simulink model "Simulation_3DOF"  (R2024a)
settings: Solver=ode4  StartTime=initial_time  StopTime=final_time  FixedStep=timestep  RelTol=1e-3
values from neighbouring files (symbols this model uses):
  gamma = 1.4    [Constants_3DOF.m]
  mass = 161.5    [Constants_3DOF.m]
  mu_earth = 3.986004418 * 10^14    (= 398600441800000)    [Constants_3DOF.m]
  r_earth = 6371.0088 * 10^3    (= 6371008.8)    [Constants_3DOF.m]
  wing_area = 0.079813    [Constants_3DOF.m]
undefined symbols (not defined in the file or in its folder): alpha, beta, c_d, c_l, rho, thrust, velocity, x, y, z
settings Model: Creator=641893  LastModifiedBy=641893

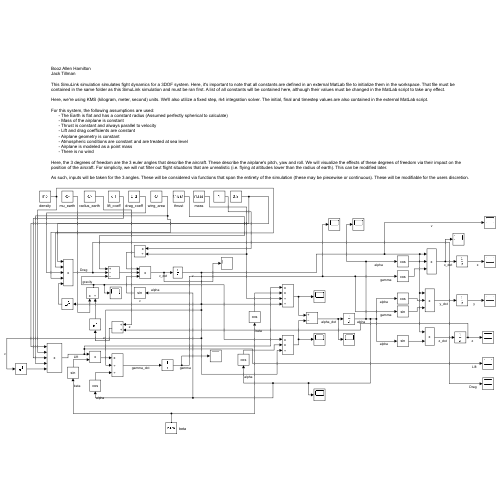
[thumbnail: Simulink's stored preview of the top-level diagram]
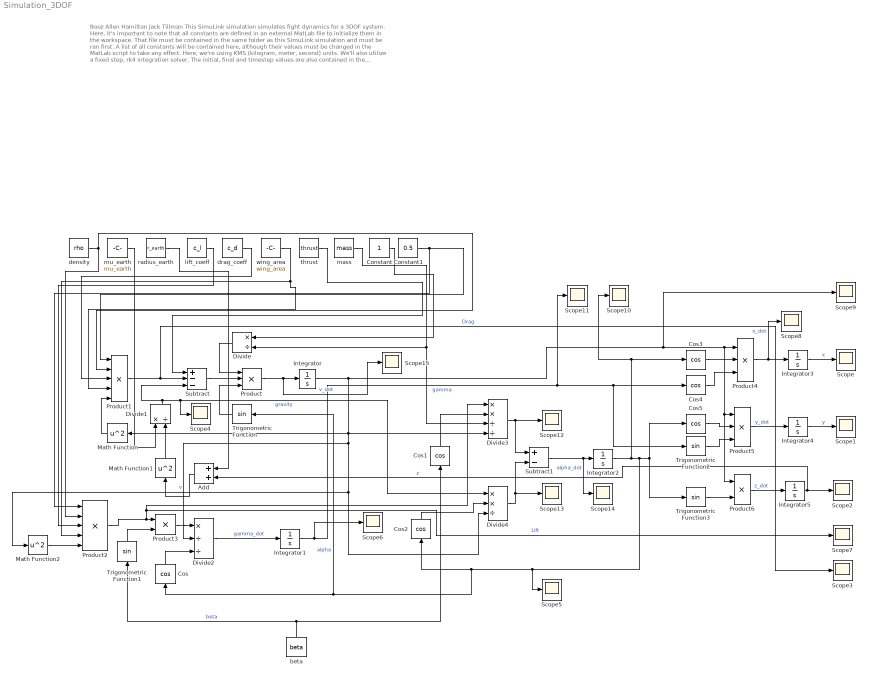
== system Simulation_3DOF ==
  note: Booz Allen Hamilton
      | Jack Tillman
      |
      | This SimuLink simulation simulates fight dynamics for a 3DOF system. Here, it's important to note that all constants are defined in an external MatLab file to initialize them in the workspace. That file must be contained in the same folder as this SimuLink simulation and must be ran first. A list of all constants will be contained here, although their values must be changed in the MatLab script to take any effect.
      |
      | Here, we're using KMS (kilogram, meter, second) units. We'll also utilize a fixed step, rk4 integration solver. The initial, final and timestep values are also contained in the external MatLab script.
      |
      | For this system, the following assumptions are used:
      | - The Earth is flat and has a constant radius (Assumed perfectly spherical to calculate)
      | - Mass of the airplane is constant
      | - Thrust is constant and always parallel to velocity
      | - Lift and drag coefficients are constant
      | - Airplane geometry is constant
      | - Atmospheric conditions are constant and are treated at sea level
      | - Airplane is modeled as a point mass
      | - There is no wind
      |
      | Here, the 3 degrees of freedom are the 3 euler angles that describe the aircraft. These describe the airplane's pitch, yaw and roll. We will visualize the effects of these degrees of freedom via their impact on the position of the aircraft. For simplicity, we will not filter out flight situations that are unrealistic (i.e. flying at altitudes lower than the radius of earth). This can be modified later.
      |
      | As such, inputs will be taken for the 3 angles. These will be considered via functions that span the entirety of the simulation (these may be piecewise or continuous). These will be modifiable for the users discretion.
  Add : Sum
  Constant : Constant
  Constant1 : Constant  Value=0.5
  Cos{,1..5} (6 alike) : Trigonometry  Operator=cos
  Divide : Product  Inputs=*/
  Divide1 : Product  Inputs=*/
  Divide2 : Product  Inputs=*//
  Divide3 : Product  Inputs=**//
  Divide4 : Product  Inputs=**/
  Integrator : Integrator  InitialCondition=velocity
  Integrator1 : Integrator  InitialCondition=gamma
  Integrator2 : Integrator  InitialCondition=alpha
  Integrator3 : Integrator  InitialCondition=x
  Integrator4 : Integrator  InitialCondition=y
  Integrator5 : Integrator  InitialCondition=z
  Math Function : Math  Operator=square
  Math Function1 : Math  Operator=square
  Math Function2 : Math  Operator=square
  Product : Product  Inputs=3
  Product1 : Product  Inputs=5
  Product2 : Product  Inputs=5
  Product3 : Product
  Product4 : Product  Inputs=3
  Product5 : Product  Inputs=3
  Product6 : Product
  Scope{,1..15} (16 alike) : Scope
  Subtract : Sum  Inputs=+--
  Subtract1 : Sum  Inputs=+-
  Trigonometric Function{,1..3} (4 alike) : Trigonometry
  beta : Constant  Value=beta
  density : Constant  Value=rho
  drag_coeff : Constant  Value=c_d
  lift_coeff : Constant  Value=c_l
  mass : Constant  Value=mass
  mu_earth : Constant  Value=mu_earth
  radius_earth : Constant  Value=r_earth
  thrust : Constant  Value=thrust
  wing_area : Constant  Value=wing_area
  wires:
  Product/1 -> Scope15/1, Integrator/1  "v_dot"
  Integrator/1 -> Scope9/1, Product6/1, Product5/1, Product4/1, Divide4/3, Math Function2/1, Divide2/2, Math Function/1, Divide3/4  "v"
  mass/1 -> Divide3/3, Divide/2
  Divide/1 -> Product/1
  Subtract/1 -> Product/2
  Trigonometric Function/1 -> Product/3
  Integrator2/1 -> Scope10/1, Cos3/1, Scope5/1, Trigonometric Function/1, Cos/1, Cos2/1, Cos5/1, Trigonometric Function3/1  "alpha"
  thrust/1 -> Subtract/1
  Product1/1 -> Scope3/1, Subtract/2  "Drag"
  Divide1/1 -> Scope4/1, Divide4/1, Subtract/3  "gravity"
  Constant/1 -> Divide/1
  Constant1/1 -> Product1/1, Product2/1
  density/1 -> Product2/2, Product1/2
  drag_coeff/1 -> Product1/3
  wing_area/1 -> Product2/4, Product1/4
  Math Function/1 -> Product1/5
  mu_earth/1 -> Divide1/1
  Math Function1/1 -> Divide1/2
  Add/1 -> Math Function1/1
  radius_earth/1 -> Add/1
  Divide2/1 -> Integrator1/1  "gamma_dot"
  lift_coeff/1 -> Product2/3
  Product2/1 -> Divide3/1, Scope7/1, Product3/1  "Lift"
  Trigonometric Function1/1 -> Product3/2
  Product3/1 -> Divide2/1
  Cos/1 -> Divide2/3
  Subtract1/1 -> Scope14/1, Integrator2/1  "alpha_dot"
  beta/1 -> Trigonometric Function1/1, Cos1/1  "beta"
  Cos1/1 -> Divide3/2
  Cos2/1 -> Divide4/2
  Divide3/1 -> Subtract1/1, Scope12/1
  Divide4/1 -> Subtract1/2, Scope13/1
  Product4/1 -> Scope8/1, Integrator3/1  "x_dot"
  Integrator3/1 -> Scope/1  "x"
  Cos3/1 -> Product4/2
  Cos4/1 -> Product4/3
  Product5/1 -> Integrator4/1  "y_dot"
  Integrator4/1 -> Scope1/1  "y"
  Cos5/1 -> Product5/2
  Trigonometric Function2/1 -> Product5/3
  Integrator1/1 -> Scope6/1, Cos4/1, Trigonometric Function2/1, Scope11/1  "gamma"
  Integrator5/1 -> Add/2, Scope2/1  "z"
  Product6/1 -> Integrator5/1  "z_dot"
  Trigonometric Function3/1 -> Product6/2
  Math Function2/1 -> Product2/5
